simulink model "simple_model"  (R2021b)
settings: Solver=ode45  StartTime=0.0  StopTime=10  RelTol=1e-5  EnableMultiTasking=on
values from neighbouring files (symbols this model uses):
  A = [0 0 1 0 ... (first row only)    [main.m]
  B = [0 ... (first row only)    [main.m]
  C = [1 0 0 0 ... (first row only)    [main.m]
  K = K_temp    [plots_assignment2.m]    (also in plots_assignment3.m)
  x_initial = [0 0 0 0]'    [main.m]    (also in tuning.m)
settings Model: Creator=magudelo  LastModifiedBy=Marius
settings SolverCC: AlgebraicLoopSolver=TrustRegion
settings DataIOCC: LimitDataPoints=on  SaveFormat=Array  SignalLoggingSaveFormat=ModelDataLogs  ReturnWorkspaceOutputs=off
settings OptimizationCC: ExpressionDepthLimit=2147483647  LifeSpan=inf
settings DebuggingCC: UnderspecifiedInitializationDetection=Classic  MergeDetectMultiDrivingBlocksExec=none  FcnCallInpInsideContextMsg=warning  AllowSymbolicDim=off  StateNameClashWarn=warning  SFUnexpectedBacktrackingDiag=warning  SFNoUnconditionalDefaultTransitionDiag=warning  SFExecutionAtInitializationDiag=none  SFMachineParentedDataDiag=warning  ArithmeticOperatorsInVariantConditions=warning
settings HardwareCC: ProdBitPerPointer=32  ProdBitPerSizeT=32  ProdBitPerPtrDiffT=32  ProdLargestAtomicFloat=None  ProdIntDivRoundTo=Undefined  ProdEndianess=Unspecified  ProdWordSize=32  ProdHWDeviceType=32-bit Generic
settings ModelReferenceCC: PropagateSignalLabelsOutOfModel=off
settings SFSimCC: SimUseLocalCustomCode=off  CustomCodeUndefinedFunction=UseInterfaceOnly
settings RTWCC: RTWUseLocalCustomCode=off
settings CodeAppCC: StateflowObjectComments=on
settings GRTTargetCC: TargetLangStandard=C89/C90 (ANSI)  CombineOutputUpdateFcns=off  GRTInterface=on
settings ConfigComp: CovMetricSettings=dw  CovSaveCumulativeToWorkspaceVar=on  CovSaveSingleToWorkspaceVar=on  CovExternalEMLEnable=off

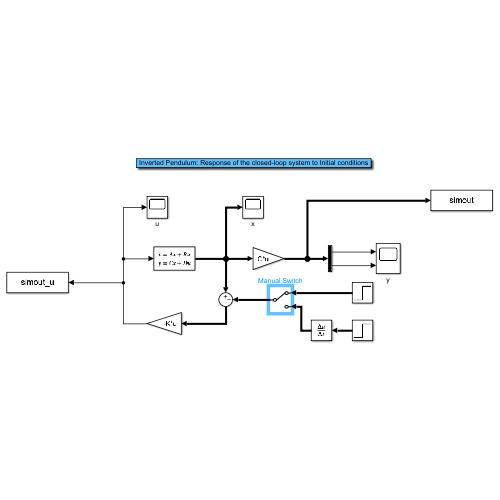
[thumbnail: Simulink's stored preview of the top-level diagram]
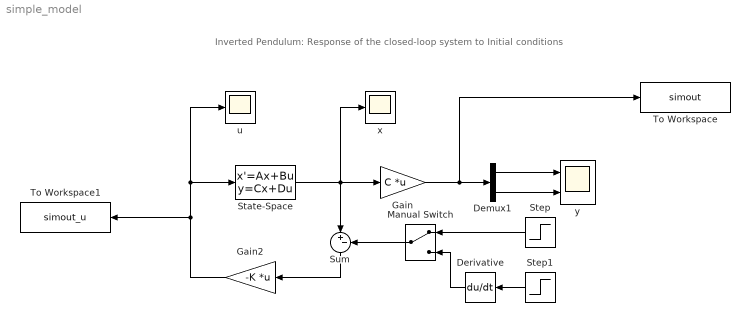
== system simple_model ==
  note: Inverted Pendulum: Response of the closed-loop system to Initial conditions
  Demux1 : Demux  Outputs=2
  Derivative : Derivative
  Gain : Gain  Gain=C  Multiplication=Matrix(K*u)
  Gain2 : Gain  Gain=-K  Multiplication=Matrix(K*u)
  Manual Switch : ManualSwitch
  State-Space : StateSpace  A=A  B=B  C=eye(4)  D=zeros(4,1)  InitialCondition=x_initial
  Step : Step  Before=[0 0 0 0]  After=[0.1 0 0 0]  SampleTime=0
  Step1 : Step  Before=[0 0 0 0]  After=[0.1 0 0 0]  SampleTime=0
  Sum : Sum  Inputs=|+-
  To Workspace : ToWorkspace  VariableName=simout  SaveFormat=Timeseries  SampleTime=-1
  To Workspace1 : ToWorkspace  VariableName=simout_u  SaveFormat=Timeseries  SampleTime=-1
  u : Scope
  x : Scope
  y : Scope  NumInputPorts=2
  wires:
  State-Space/1 -> Gain/1, Sum/1, x/1
  Gain/1 -> To Workspace/1, Demux1/1
  Gain2/1 -> To Workspace1/1, u/1, State-Space/1
  Demux1/1 -> y/1
  Demux1/2 -> y/2
  Sum/1 -> Gain2/1
  Manual Switch/1 -> Sum/2
  Step/1 -> Manual Switch/1
  Step1/1 -> Derivative/1
  Derivative/1 -> Manual Switch/2
